simulink model "uav_closed_loop_v5"  (R2016a)
settings: Solver=VariableStepAuto  StartTime=0.0  StopTime=10.0  RelTol=1e-3
values from neighbouring files (symbols this model uses):
  initialState = zeros(1,nPreviousStatesArray(iIndividual))    [uav_evaluation_function.m]
  phiMax = UavParam.phiMax    [uav_evaluation_function.m]
  phiMin = UavParam.phiMin    [uav_evaluation_function.m]
  psiMax = UavParam.psiMax    [uav_evaluation_function.m]
  psiMin = UavParam.psiMin    [uav_evaluation_function.m]
  thetaMax = UavParam.thetaMax    [uav_evaluation_function.m]
  thetaMin = UavParam.thetaMin    [uav_evaluation_function.m]
  xMax = UavParam.xMax    [uav_evaluation_function.m]
  xMin = UavParam.xMin    [uav_evaluation_function.m]
  yMax = UavParam.yMax    [uav_evaluation_function.m]
  yMin = UavParam.yMin    [uav_evaluation_function.m]
  zMax = UavParam.zMax    [uav_evaluation_function.m]
  zMin = UavParam.zMin    [uav_evaluation_function.m]
undefined symbols (not defined in the file or in its folder): fullLogging, g, I, loggingSampleTime, m, maxViolationPhi, maxViolationPsi, maxViolationTheta, maxViolationX, maxViolationY, maxViolationZ, nMotors, omega1Max, omega1Min, omega2Max, omega2Min, omega3Max, omega3Min, omega4Max, omega4Min, phiDesiredMax, phiDesiredMin, pMax, pMin, psiDesiredMax, psiDesiredMin, qMax, qMin, rMax, rMin, thetaDesiredMax, thetaDesiredMin, udotMax, udotMin, uMax, uMin, VaMax, VaMin, vdotMax, vdotMin, vMax, vMin, wdotMax, wdotMin, wMax, wMin, xDesiredMax, xDesiredMin, yDesiredMax, yDesiredMin, zDesiredMax, zDesiredMin
libraries: uav_library x32, simulink x6, neural x1
settings Model: Creator=Maxence  LastModifiedBy=Maxence

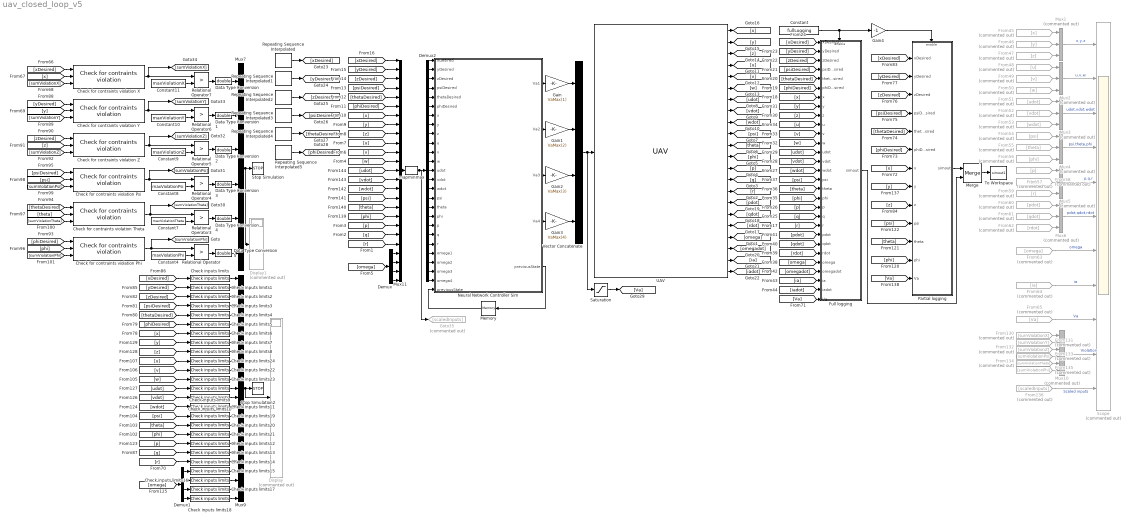
== system uav_closed_loop_v5 ==
  Check for contraints violation Phi : uav_library/Check for contraints violation  violationFactor=violationFactorPhi  lowerQTol=lowerPhiTol  upperQTol=upperPhiTol  currentTimeThreshold=currentTimeThresholdPhi
  Check for contraints violation Psi : uav_library/Check for contraints violation  violationFactor=violationFactorPsi  lowerQTol=lowerPsiTol  upperQTol=upperPsiTol  currentTimeThreshold=currentTimeThresholdPsi
  Check for contraints violation Theta : uav_library/Check for contraints violation  violationFactor=violationFactorTheta  lowerQTol=lowerThetaTol  upperQTol=upperThetaTol  currentTimeThreshold=currentTimeThresholdTheta
  Check for contraints violation X : uav_library/Check for contraints violation  violationFactor=violationFactorX  lowerQTol=lowerXTol  upperQTol=upperXTol  currentTimeThreshold=currentTimeThresholdX
  Check for contraints violation Y : uav_library/Check for contraints violation  violationFactor=violationFactorY  lowerQTol=lowerYTol  upperQTol=upperYTol  currentTimeThreshold=currentTimeThresholdY
  Check for contraints violation Z : uav_library/Check for contraints violation  violationFactor=violationFactorZ  lowerQTol=lowerZTol  upperQTol=upperZTol  currentTimeThreshold=currentTimeThresholdZ
  Check inputs limits : uav_library/Check inputs limits  qMin=xDesiredMin  qMax=xDesiredMax
  Check inputs limits1 : uav_library/Check inputs limits  qMin=yDesiredMin  qMax=yDesiredMax
  Check inputs limits10 : uav_library/Check inputs limits  qMin=vdotMin  qMax=vdotMax
  Check inputs limits11 : uav_library/Check inputs limits  qMin=wdotMin  qMax=wdotMax
  Check inputs limits12 : uav_library/Check inputs limits  qMin=pMin  qMax=pMax
  Check inputs limits13 : uav_library/Check inputs limits  qMin=qMin  qMax=qMax
  Check inputs limits14 : uav_library/Check inputs limits  qMin=rMin  qMax=rMax
  Check inputs limits15 : uav_library/Check inputs limits  qMin=omega1Min  qMax=omega1Max
  Check inputs limits16 : uav_library/Check inputs limits  qMin=omega2Min  qMax=omega2Max
  Check inputs limits17 : uav_library/Check inputs limits  qMin=omega3Min  qMax=omega3Max
  Check inputs limits18 : uav_library/Check inputs limits  qMin=omega4Min  qMax=omega4Max
  Check inputs limits19 : uav_library/Check inputs limits  qMin=psiMin  qMax=psiMax
  Check inputs limits2 : uav_library/Check inputs limits  qMin=zDesiredMin  qMax=zDesiredMax
  Check inputs limits20 : uav_library/Check inputs limits  qMin=thetaMin  qMax=thetaMax
  Check inputs limits21 : uav_library/Check inputs limits  qMin=phiMin  qMax=phiMax
  Check inputs limits22 : uav_library/Check inputs limits  qMin=vMin  qMax=vMax
  Check inputs limits23 : uav_library/Check inputs limits  qMin=wMin  qMax=wMax
  Check inputs limits24 : uav_library/Check inputs limits  qMin=uMin  qMax=uMax
  Check inputs limits3 : uav_library/Check inputs limits  qMin=psiDesiredMin  qMax=psiDesiredMax
  Check inputs limits4 : uav_library/Check inputs limits  qMin=thetaDesiredMin  qMax=thetaDesiredMax
  Check inputs limits5 : uav_library/Check inputs limits  qMin=phiDesiredMin  qMax=phiDesiredMax
  Check inputs limits6 : uav_library/Check inputs limits  qMin=xMin  qMax=xMax
  Check inputs limits7 : uav_library/Check inputs limits  qMin=yMin  qMax=yMax
  Check inputs limits8 : uav_library/Check inputs limits  qMin=zMin  qMax=zMax
  Check inputs limits9 : uav_library/Check inputs limits  qMin=udotMin  qMax=udotMax
  Constant : Constant  Value=fullLogging
  Constant10 : Constant  Value=maxViolationY
  Constant11 : Constant  Value=maxViolationX
  Constant4 : Constant  Value=maxViolationPhi
  Constant7 : Constant  Value=maxViolationTheta
  Constant8 : Constant  Value=maxViolationPsi
  Constant9 : Constant  Value=maxViolationZ
  Data Type Conversion{,1..5} (6 alike) : DataTypeConversion  OutDataTypeStr=double
  Demux : Demux
  Demux1 : Demux
  Demux2 : Demux  Outputs=25
  Display : Display  Commented=on
  Display1 : Display  Commented=on
  From130 : From  Commented=on  GotoTag=sumViolationX
  From131 : From  Commented=on  GotoTag=sumViolationY
  From132 : From  Commented=on  GotoTag=sumViolationZ
  From133 : From  Commented=on  GotoTag=sumViolationPsi
  From134 : From  Commented=on  GotoTag=sumViolationTheta
  From135 : From  Commented=on  GotoTag=sumViolationPhi
  From136 : From  Commented=on  GotoTag=scaledInputs
  From45 : From  Commented=on  GotoTag=x
  From46 : From  Commented=on  GotoTag=y
  From47 : From  Commented=on  GotoTag=z
  From48 : From  Commented=on  GotoTag=u
  From49 : From  Commented=on  GotoTag=v
  From50 : From  Commented=on  GotoTag=w
  From51 : From  Commented=on  GotoTag=udot
  From52 : From  Commented=on  GotoTag=vdot
  From53 : From  Commented=on  GotoTag=wdot
  From54 : From  Commented=on  GotoTag=psi
  From55 : From  Commented=on  GotoTag=theta
  From56 : From  Commented=on  GotoTag=phi
  From57 : From  Commented=on  GotoTag=p
  From58 : From  Commented=on  GotoTag=q
  From59 : From  Commented=on  GotoTag=r
  From60 : From  Commented=on  GotoTag=pdot
  From61 : From  Commented=on  GotoTag=qdot
  From62 : From  Commented=on  GotoTag=rdot
  From63 : From  Commented=on  GotoTag=omega
  From64 : From  Commented=on  GotoTag=ia
  From65 : From  Commented=on  GotoTag=Va
  Full logging : Subsystem
  Gain : Gain  Gain=VaMax(1)
  Gain1 : Gain  Gain=VaMax(2)
  Gain2 : Gain  Gain=VaMax(3)
  Gain3 : Gain  Gain=VaMax(4)
  Gain4 : Gain  Gain=-1
  Goto35 : Goto  Commented=on  GotoTag=scaledInputs
  Memory : Memory  X0=initialState
  Merge : Merge
  Mux{1..6} (6 alike) : Mux  Commented=on  Inputs=3
  Mux10 : Mux  Commented=on  Inputs=6
  Mux11 : Mux  Inputs=25
  Mux7 : Mux  Inputs=6
  Mux9 : Mux  Inputs=25
  Neural Network Controller Sim : MATLAB Function  TreatAsAtomicUnit=on
      settings: RTWSystemCode=Nonreusable function
  Partial logging : Subsystem
  Relational Operator{,3..7} (6 alike) : RelationalOperator  Operator=>  OutDataTypeStr=boolean  ZeroCross=off
  Repeating Sequence Interpolated : simulink/Sources/Repeating Sequence Interpolated  OutValues=XDesired.val'  TimeValues=XDesired.t'  LookUpMeth=Interpolation-Use End Values  tsamp=0.01  OutMin=[]  OutMax=[]  OutDataTypeStr=double  OutputDataTypeScalingMode=double  OutDataType=fixdt(0,8)  OutScaling=2^-10
  Repeating Sequence Interpolated1 : simulink/Sources/Repeating Sequence Interpolated  OutValues=YDesired.val'  TimeValues=YDesired.t'  LookUpMeth=Interpolation-Use End Values  tsamp=0.01  OutMin=[]  OutMax=[]  OutDataTypeStr=double  OutputDataTypeScalingMode=double  OutDataType=fixdt(0,8)  OutScaling=2^-10
  Repeating Sequence Interpolated2 : simulink/Sources/Repeating Sequence Interpolated  OutValues=ZDesired.val'  TimeValues=ZDesired.t'  LookUpMeth=Interpolation-Use End Values  tsamp=0.01  OutMin=[]  OutMax=[]  OutDataTypeStr=double  OutputDataTypeScalingMode=double  OutDataType=fixdt(0,8)  OutScaling=2^-10
  Repeating Sequence Interpolated3 : simulink/Sources/Repeating Sequence Interpolated  OutValues=PsiDesired.val'  TimeValues=PsiDesired.t'  LookUpMeth=Interpolation-Use End Values  tsamp=0.01  OutMin=[]  OutMax=[]  OutDataTypeStr=double  OutputDataTypeScalingMode=double  OutDataType=fixdt(0,8)  OutScaling=2^-10
  Repeating Sequence Interpolated4 : simulink/Sources/Repeating Sequence Interpolated  OutValues=ThetaDesired.val'  TimeValues=ThetaDesired.t'  LookUpMeth=Interpolation-Use End Values  tsamp=0.01  OutMin=[]  OutMax=[]  OutDataTypeStr=double  OutputDataTypeScalingMode=double  OutDataType=fixdt(0,8)  OutScaling=2^-10
  Repeating Sequence Interpolated5 : simulink/Sources/Repeating Sequence Interpolated  OutValues=PhiDesired.val'  TimeValues=PhiDesired.t'  LookUpMeth=Interpolation-Use End Values  tsamp=0.01  OutMin=[]  OutMax=[]  OutDataTypeStr=double  OutputDataTypeScalingMode=double  OutDataType=fixdt(0,8)  OutScaling=2^-10
  Saturation : Saturate  UpperLimit=VaMax  LowerLimit=VaMin
  Scope : Scope  Commented=on  NumInputPorts=11
  Stop Simulation : Stop
  Stop Simulation2 : Stop
  To Workspace : ToWorkspace  VariableName=simout1  SaveFormat=Structure With Time  SampleTime=loggingSampleTime
  UAV : uav_library/UAV  g=g  activateMast=off  config=X4  nMotors=nMotors  m=m  I=I  PP=PP  Ra=Ra  La=La  ke=ke  km=km  kD=kD  Jm=Jm  Bm=Bm  kT=kT  VaMin=VaMin  VaMax=VaMax  omegaInitial=omegaInitial  omegaDelay=omegaDelay  iaInitial=iaInitial  iaDelay=iaDelay  vPtInitial=vPtInitial  vPtDelay=vPtDelay  xPInitial=xPInitial  xPDelay=xPDelay  omegabtInitial=omegabtInitial  omegabtDelay=omegabtDelay  eulerZYXInitial=eulerZYXInitial  eulerZYXDelay=eulerZYXDelay
  Vector Concatenate : Concatenate  NumInputs=4
  mapminmax : neural/Processing Functions/mapminmax  xmin=[xDesiredMin; yDesiredMin; zDesiredMin; psiDesiredMin; thetaDesiredMin; phiDesiredMin; xMin; yMin; zMin; uMin; vMin; wMin; udotMin; vdotMin; wdotMin; psiMin; thetaMin; phiMin; pMin; qMin; rMin; omega1Min; omega2Min; omega3Min; omega4Min]  xmax=[xDesiredMax; yDesiredMax; zDesiredMax; psiDesiredMax; thetaDesiredMax; phiDesiredMax; xMax; yMax; zMax; uMax; vMax; wMax; udotMax; vdotMax; wdotMax; psiMax; thetaMax; phiMax; pMax; qMax; rMax; omega1Max; omega2Max; omega3Max; omega4Max]  ymin=-1  ymax=+1
  wires:
  Vector Concatenate/1 -> Saturation/1, UAV/1
  Neural Network Controller Sim/1(Va1) -> Gain/1
  UAV/19 -> [omega]
  [omega] -> Demux/1
  UAV/15 -> [r]
  UAV/14 -> [q]
  UAV/13 -> [p]
  UAV/12 -> [phi]
  UAV/11 -> [theta]
  UAV/10 -> [psi]
  UAV/7 -> [udot]
  UAV/8 -> [vdot]
  UAV/9 -> [wdot]
  UAV/4 -> [u]
  UAV/5 -> [v]
  UAV/6 -> [w]
  UAV/3 -> [z]
  UAV/2 -> [y]
  UAV/1 -> [x]
  [wdot] -> Mux11/15
  [vdot] -> Mux11/14
  [udot] -> Mux11/13
  [w] -> Mux11/12
  [v] -> Mux11/11
  [u] -> Mux11/10
  [z] -> Mux11/9
  [y] -> Mux11/8
  [x] -> Mux11/7
  [phiDesired] -> Mux11/6
  [thetaDesired] -> Mux11/5
  [psiDesired] -> Mux11/4
  [zDesired] -> Mux11/3
  [yDesired] -> Mux11/2
  [xDesired] -> Mux11/1
  UAV/16 -> [pdot]
  UAV/17 -> [qdot]
  UAV/18 -> [rdot]
  UAV/20 -> [omegadot]
  UAV/21 -> [ia]
  UAV/22 -> [iadot]
  Repeating Sequence Interpolated/1 -> [xDesired]
  Repeating Sequence Interpolated1/1 -> [yDesired]
  Repeating Sequence Interpolated2/1 -> [zDesired]
  Repeating Sequence Interpolated3/1 -> [psiDesired]
  Repeating Sequence Interpolated4/1 -> [thetaDesired]
  Repeating Sequence Interpolated5/1 -> [phiDesired]
  Neural Network Controller Sim/5(previousState) -> Memory/1
  Memory/1 -> Neural Network Controller Sim/26("previousState ")
  From45/1 -> Mux1/1
  From46/1 -> Mux1/2
  From47/1 -> Mux1/3
  From48/1 -> Mux2/1
  From49/1 -> Mux2/2
  From50/1 -> Mux2/3
  From51/1 -> Mux3/1
  From52/1 -> Mux3/2
  From53/1 -> Mux3/3
  From54/1 -> Mux4/1
  From55/1 -> Mux4/2
  From56/1 -> Mux4/3
  From58/1 -> Mux5/2
  From59/1 -> Mux5/3
  From57/1 -> Mux5/1
  From60/1 -> Mux6/1
  From61/1 -> Mux6/2
  From62/1 -> Mux6/3
  From63/1 -> Scope/7  "omega"
  Mux1/1 -> Scope/1  "x,y,z"
  Mux2/1 -> Scope/2  "u,v,w"
  Mux3/1 -> Scope/3  "udot,vdot,wdot"
  Mux4/1 -> Scope/4  "psi,theta,phi"
  Mux5/1 -> Scope/5  "p,q,r"
  Mux6/1 -> Scope/6  "pdot,qdot,rdot"
  From64/1 -> Scope/8  "ia"
  From65/1 -> Scope/9  "Va"
  Constant4/1 -> Relational Operator/2
  Check for contraints violation Phi/1 -> [sumViolationPhi], Relational Operator/1
  Constant7/1 -> Relational Operator3/2
  Check for contraints violation Theta/1 -> [sumViolationTheta], Relational Operator3/1
  Constant8/1 -> Relational Operator4/2
  Check for contraints violation Psi/1 -> [sumViolationPsi], Relational Operator4/1
  Constant9/1 -> Relational Operator5/2
  Check for contraints violation Z/1 -> [sumViolationZ], Relational Operator5/1
  Constant10/1 -> Relational Operator6/2
  Check for contraints violation Y/1 -> [sumViolationY], Relational Operator6/1
  Constant11/1 -> Relational Operator7/2
  Check for contraints violation X/1 -> [sumViolationX], Relational Operator7/1
  Relational Operator7/1 -> Data Type Conversion/1
  Relational Operator6/1 -> Data Type Conversion1/1
  Mux7/1 -> Display1/1, Stop Simulation/1
  Data Type Conversion1/1 -> Mux7/2
  Data Type Conversion/1 -> Mux7/1
  Relational Operator5/1 -> Data Type Conversion2/1
  Data Type Conversion2/1 -> Mux7/3
  Relational Operator4/1 -> Data Type Conversion3/1
  Data Type Conversion3/1 -> Mux7/4
  Relational Operator3/1 -> Data Type Conversion4/1
  Data Type Conversion4/1 -> Mux7/5
  Relational Operator/1 -> Data Type Conversion5/1
  Data Type Conversion5/1 -> Mux7/6
  [xDesired] -> Check for contraints violation X/1
  [x] -> Check for contraints violation X/2
  [sumViolationX] -> Check for contraints violation X/3
  [yDesired] -> Check for contraints violation Y/1
  [y] -> Check for contraints violation Y/2
  [sumViolationY] -> Check for contraints violation Y/3
  [zDesired] -> Check for contraints violation Z/1
  [z] -> Check for contraints violation Z/2
  [sumViolationZ] -> Check for contraints violation Z/3
  [psiDesired] -> Check for contraints violation Psi/1
  [psi] -> Check for contraints violation Psi/2
  [sumViolationPsi] -> Check for contraints violation Psi/3
  [thetaDesired] -> Check for contraints violation Theta/1
  [theta] -> Check for contraints violation Theta/2
  [sumViolationTheta] -> Check for contraints violation Theta/3
  [phiDesired] -> Check for contraints violation Phi/1
  [phi] -> Check for contraints violation Phi/2
  [sumViolationPhi] -> Check for contraints violation Phi/3
  Gain/1 -> Vector Concatenate/1
  Gain1/1 -> Vector Concatenate/2
  Gain2/1 -> Vector Concatenate/3
  Gain3/1 -> Vector Concatenate/4
  Merge/1 -> To Workspace/1
  Demux2/1 -> Neural Network Controller Sim/1(xDesired)
  Demux2/2 -> Neural Network Controller Sim/2(yDesired)
  Demux2/3 -> Neural Network Controller Sim/3(zDesired)
  Demux2/4 -> Neural Network Controller Sim/4(psiDesired)
  Demux2/5 -> Neural Network Controller Sim/5(thetaDesired)
  Demux2/6 -> Neural Network Controller Sim/6(phiDesired)
  Demux2/7 -> Neural Network Controller Sim/7(x)
  Demux2/8 -> Neural Network Controller Sim/8(y)
  Demux2/9 -> Neural Network Controller Sim/9(z)
  Demux1/1 -> Check inputs limits15/1
  Demux1/2 -> Check inputs limits16/1
  Demux1/4 -> Check inputs limits18/1
  [omega] -> Demux1/1
  [r] -> Check inputs limits14/1
  [q] -> Check inputs limits13/1
  [p] -> Check inputs limits12/1
  [wdot] -> Check inputs limits11/1
  [vdot] -> Check inputs limits10/1
  [udot] -> Check inputs limits9/1
  [z] -> Check inputs limits8/1
  [y] -> Check inputs limits7/1
  [x] -> Check inputs limits6/1
  [phiDesired] -> Check inputs limits5/1
  [thetaDesired] -> Check inputs limits4/1
  [psiDesired] -> Check inputs limits3/1
  [zDesired] -> Check inputs limits2/1
  [yDesired] -> Check inputs limits1/1
  [xDesired] -> Check inputs limits/1
  Demux1/3 -> Check inputs limits17/1
  Check inputs limits/1 -> Mux9/1
  Check inputs limits1/1 -> Mux9/2
  Check inputs limits2/1 -> Mux9/3
  Check inputs limits3/1 -> Mux9/4
  Check inputs limits4/1 -> Mux9/5
  Check inputs limits5/1 -> Mux9/6
  Check inputs limits6/1 -> Mux9/7
  Check inputs limits7/1 -> Mux9/8
  Check inputs limits8/1 -> Mux9/9
  Check inputs limits24/1 -> Mux9/10
  Check inputs limits22/1 -> Mux9/11
  Check inputs limits23/1 -> Mux9/12
  Check inputs limits9/1 -> Mux9/13
  Check inputs limits10/1 -> Mux9/14
  Check inputs limits11/1 -> Mux9/15
  Mux9/1 -> Display/1, Stop Simulation2/1
  Mux10/1 -> Scope/10  "Violation"
  From130/1 -> Mux10/1
  From131/1 -> Mux10/2
  From132/1 -> Mux10/3
  From133/1 -> Mux10/4
  From134/1 -> Mux10/5
  From135/1 -> Mux10/6
  From136/1 -> Scope/11  "Scaled inputs"
  Mux11/1 -> mapminmax/1
  Saturation/1 -> [Va]
  [xDesired] -> Full logging/1(xDesired)
  [yDesired] -> Full logging/2(yDesired)
  [zDesired] -> Full logging/3(zDesired)
  [psiDesired] -> Full logging/4(psiDesired)
  [thetaDesired] -> Full logging/5(thetaDesired)
  [phiDesired] -> Full logging/6(phiDesired)
  [x] -> Full logging/7(x)
  [y] -> Full logging/8(y)
  [z] -> Full logging/9(z)
  [u] -> Full logging/10(u)
  [v] -> Full logging/11(v)
  [w] -> Full logging/12(w)
  [udot] -> Full logging/13(udot)
  [vdot] -> Full logging/14(vdot)
  [wdot] -> Full logging/15(wdot)
  [psi] -> Full logging/16(psi)
  [theta] -> Full logging/17(theta)
  [phi] -> Full logging/18(phi)
  [p] -> Full logging/19(p)
  [q] -> Full logging/20(q)
  [r] -> Full logging/21(r)
  [pdot] -> Full logging/22(pdot)
  [qdot] -> Full logging/23(qdot)
  [rdot] -> Full logging/24(rdot)
  [omega] -> Full logging/25(omega)
  [omegadot] -> Full logging/26(omegadot)
  [ia] -> Full logging/27(ia)
  [iadot] -> Full logging/28(iadot)
  Full logging/1(simout) -> Merge/2
  [xDesired] -> Partial logging/1(xDesired)
  [yDesired] -> Partial logging/2(yDesired)
  [zDesired] -> Partial logging/3(zDesired)
  [psiDesired] -> Partial logging/4(psiDesired)
  [thetaDesired] -> Partial logging/5(thetaDesired)
  [phiDesired] -> Partial logging/6(phiDesired)
  [x] -> Partial logging/7(x)
  [y] -> Partial logging/8(y)
  [z] -> Partial logging/9(z)
  [psi] -> Partial logging/10(psi)
  [theta] -> Partial logging/11(theta)
  [phi] -> Partial logging/12(phi)
  Partial logging/1(simout) -> Merge/1
  Constant/1 -> Gain4/1, Full logging/Enable
  Gain4/1 -> Partial logging/Enable
  [Va] -> Full logging/29(Va)
  [Va] -> Partial logging/13(Va)
  Demux/2 -> Mux11/23
  Demux/1 -> Mux11/22
  Demux/3 -> Mux11/24
  Demux/4 -> Mux11/25
  [r] -> Mux11/21
  [q] -> Mux11/20
  [p] -> Mux11/19
  [phi] -> Mux11/18
  [theta] -> Mux11/17
  [psi] -> Mux11/16
  Demux2/10 -> Neural Network Controller Sim/10(u)
  Demux2/25 -> Neural Network Controller Sim/25(omega4)
  Demux2/24 -> Neural Network Controller Sim/24(omega3)
  Demux2/23 -> Neural Network Controller Sim/23(omega2)
  Demux2/22 -> Neural Network Controller Sim/22(omega1)
  Demux2/21 -> Neural Network Controller Sim/21(r)
  Demux2/20 -> Neural Network Controller Sim/20(q)
  Demux2/19 -> Neural Network Controller Sim/19(p)
  Demux2/18 -> Neural Network Controller Sim/18(phi)
  Demux2/17 -> Neural Network Controller Sim/17(theta)
  Demux2/16 -> Neural Network Controller Sim/16(psi)
  Demux2/15 -> Neural Network Controller Sim/15(wdot)
  Demux2/14 -> Neural Network Controller Sim/14(vdot)
  Demux2/13 -> Neural Network Controller Sim/13(udot)
  Demux2/12 -> Neural Network Controller Sim/12(w)
  Demux2/11 -> Neural Network Controller Sim/11(v)
  Neural Network Controller Sim/4(Va4) -> Gain3/1
  Neural Network Controller Sim/3(Va3) -> Gain2/1
  Neural Network Controller Sim/2(Va2) -> Gain1/1
  mapminmax/1 -> Goto35/1, Demux2/1
  Check inputs limits18/1 -> Mux9/25
  Check inputs limits17/1 -> Mux9/24
  Check inputs limits16/1 -> Mux9/23
  Check inputs limits15/1 -> Mux9/22
  Check inputs limits14/1 -> Mux9/21
  Check inputs limits13/1 -> Mux9/20
  Check inputs limits12/1 -> Mux9/19
  [phi] -> Check inputs limits21/1
  [theta] -> Check inputs limits20/1
  [psi] -> Check inputs limits19/1
  Check inputs limits19/1 -> Mux9/16
  Check inputs limits20/1 -> Mux9/17
  Check inputs limits21/1 -> Mux9/18
  [w] -> Check inputs limits23/1
  [v] -> Check inputs limits22/1
  [u] -> Check inputs limits24/1

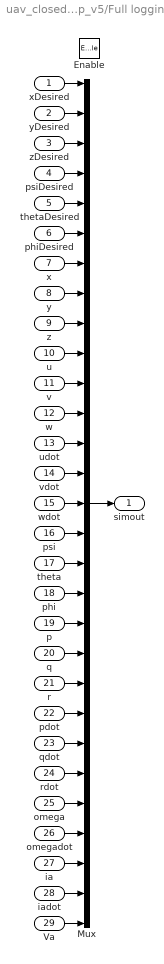
== system uav_closed_loop_v5/Full logging ==
  xDesired : Inport
  yDesired : Inport  Port=2
  zDesired : Inport  Port=3
  psiDesired : Inport  Port=4
  thetaDesired : Inport  Port=5
  phiDesired : Inport  Port=6
  x : Inport  Port=7
  y : Inport  Port=8
  z : Inport  Port=9
  u : Inport  Port=10
  v : Inport  Port=11
  w : Inport  Port=12
  udot : Inport  Port=13
  vdot : Inport  Port=14
  wdot : Inport  Port=15
  psi : Inport  Port=16
  theta : Inport  Port=17
  phi : Inport  Port=18
  p : Inport  Port=19
  q : Inport  Port=20
  r : Inport  Port=21
  pdot : Inport  Port=22
  qdot : Inport  Port=23
  rdot : Inport  Port=24
  omega : Inport  Port=25
  omegadot : Inport  Port=26
  ia : Inport  Port=27
  iadot : Inport  Port=28
  Va : Inport  Port=29
  Enable : EnablePort  StatesWhenEnabling=reset
  Mux : Mux  Inputs=29
  simout : Outport
  wires:
  pdot/1 -> Mux/22
  Mux/1 -> simout/1
  qdot/1 -> Mux/23
  rdot/1 -> Mux/24
  zDesired/1 -> Mux/3
  phiDesired/1 -> Mux/6
  udot/1 -> Mux/13
  v/1 -> Mux/11
  yDesired/1 -> Mux/2
  xDesired/1 -> Mux/1
  y/1 -> Mux/8
  w/1 -> Mux/12
  wdot/1 -> Mux/15
  x/1 -> Mux/7
  r/1 -> Mux/21
  omega/1 -> Mux/25
  omegadot/1 -> Mux/26
  ia/1 -> Mux/27
  q/1 -> Mux/20
  iadot/1 -> Mux/28
  phi/1 -> Mux/18
  psiDesired/1 -> Mux/4
  u/1 -> Mux/10
  vdot/1 -> Mux/14
  thetaDesired/1 -> Mux/5
  psi/1 -> Mux/16
  z/1 -> Mux/9
  p/1 -> Mux/19
  theta/1 -> Mux/17
  Va/1 -> Mux/29

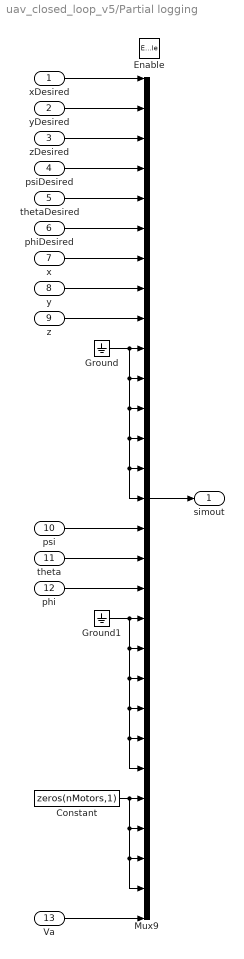
== system uav_closed_loop_v5/Partial logging ==
  xDesired : Inport
  yDesired : Inport  Port=2
  zDesired : Inport  Port=3
  psiDesired : Inport  Port=4
  thetaDesired : Inport  Port=5
  phiDesired : Inport  Port=6
  x : Inport  Port=7
  y : Inport  Port=8
  z : Inport  Port=9
  psi : Inport  Port=10
  theta : Inport  Port=11
  phi : Inport  Port=12
  Va : Inport  Port=13
  Enable : EnablePort  StatesWhenEnabling=reset
  Constant : Constant  Value=zeros(nMotors,1)
  Ground : Ground
  Ground1 : Ground
  Mux9 : Mux  Inputs=29
  simout : Outport
  wires:
  theta/1 -> Mux9/17
  phi/1 -> Mux9/18
  y/1 -> Mux9/8
  xDesired/1 -> Mux9/1
  yDesired/1 -> Mux9/2
  x/1 -> Mux9/7
  thetaDesired/1 -> Mux9/5
  zDesired/1 -> Mux9/3
  Ground/1 -> Mux9/15, Mux9/14, Mux9/13, Mux9/12, Mux9/11, Mux9/10
  psiDesired/1 -> Mux9/4
  phiDesired/1 -> Mux9/6
  z/1 -> Mux9/9
  psi/1 -> Mux9/16
  Mux9/1 -> simout/1
  Ground1/1 -> Mux9/23, Mux9/24, Mux9/22, Mux9/21, Mux9/20, Mux9/19
  Constant/1 -> Mux9/26, Mux9/27, Mux9/28, Mux9/25
  Va/1 -> Mux9/29

== matlab function uav_closed_loop_v5/Neural Network Controller Sim ==
  data: xDesired input; Va1 output; yDesired input; zDesired input; Va2 output; Va3 output; Va4 output; psiDesired input; thetaDesired input; phiDesired input; x input; y input; z input; u input; v input; w input; udot input; vdot input; wdot input; previousState output; psi input; theta input; phi input; p input; q input; r input; omega1 input; omega2 input; omega3 input; omega4 input; previousState input
function [Va1, Va2, Va3, Va4, previousState] = ...
    neural_network_controller_sim(...
    xDesired, yDesired, zDesired, ...
    psiDesired, thetaDesired, phiDesired, ...
    x, y, z, ...
    u, v, w, ...
    udot, vdot, wdot, ...
    psi, theta, phi, ...
    p, q, r, ...
    omega1, omega2, omega3, omega4, ...
    previousState)
%#codegen

% Evaluate neural network
[Va1, Va2, Va3, Va4, previousState] = uav_nn_controller(...
    xDesired, yDesired, zDesired, ...
    psiDesired, thetaDesired, phiDesired, ...
    x, y, z, ...
    u, v, w, ...
    udot, vdot, wdot, ...
    psi, theta, phi, ...
    p, q, r, ...
    omega1, omega2, omega3, omega4, previousState);
